simulink model "FFM_Punch"  (R2017a)
settings: Solver=ode3  StartTime=0.0  StopTime=timesteps  FixedStep=data.SIM.Ts  RelTol=1e-3  EnableMultiTasking=on
values from neighbouring files (symbols this model uses):
  data =     [dakota_config.mat]
  downshift_map = data.TCU.upshift.veh_spd_default    [Simulation_results.m]
  upshift_map = data.TCU.upshift.veh_spd_default    [Simulation_results.m]
undefined symbols (not defined in the file or in its folder): air_density, Cd, DiscIntNeverNeededParam, fr_crankshaft, fr_speed_values, g, i_FD, ICE, Low_Ratio, M_Eng_Max, M_Eng_Max_Max, M_Eng_Max_Rpm, mt2m_f, mu_Roll_C0, mu_Roll_C1, mu_Roll_C2, Mv, n_Idle_Eng, Overdrive_Ratio, Re, S_eff_drag, Ts
(part 4 of 15)

== system FFM_Punch/Vehicle/Subsystem ==
  v_veh : Inport  Tag=Controls_Lib  Description=Inp  Interpolate=off
  AddSub : Sum  Tag=Controls_Lib  Description=AddSub  Inputs=+++  CollapseDim=CollapseDim  AccumDataTypeStr=single  OutMin=OutMin  OutMax=OutMax  OutDataTypeStr=single  RndMeth=Nearest  SampleTime=SampleTime  InputSameDT=on  mask(AddSub){IconShape=rectangular, Inputs=+++, CollapseMode=All dimensions, CollapseDim=1, SampleTime=-1, InputSameDT=on, AccumDataTypeStr=single, OutMin=[], OutMax=[], OutDataTypeStr=single, LockScale=off, RndMeth=Nearest, SaturateOnIntegerOverflow=off}
      mask prompts: IconShape "Icon shape:"; Inputs "List of signs:"; CollapseMode "Sum over:"; CollapseDim "Dimension:"; SampleTime "Sample time (-1 for inherited):"; InputSameDT "Require all inputs to have the same data type"; AccumDataTypeStr "Accumulator data type:"; OutMin "Output minimum:"; OutMax "Output maximum:"; OutDataTypeStr "Output data type:"; LockScale "Lock data type settings against changes by the fixed-point tools"; RndMeth "Integer rounding mode:"; SaturateOnIntegerOverflow "Saturate on integer overflow"
      mask help:
      | Add or subtract inputs.  Specify one of the following:
      | a) string containing + or - for each input port, | for spacer between ports (e.g. ++|-|++)
      | b) scalar, >= 1, specifies the number of input ports to be summed.
      | When there is only one input port, add or subtract elements over all dimensions or one specified dimension
      mask Help: web([fileparts(which('Lib_built')) filesep 'hlp' filesep 'lib_AddSub' '.html'], '-helpbrowser')
      mask TypeOptions IconShape: IconShape
      mask TypeOptions Inputs: Inputs
      mask TypeOptions CollapseMode: CollapseMode
      mask TypeOptions CollapseDim: CollapseDim
      mask TypeOptions SampleTime: SampleTime
      mask TypeOptions InputSameDT: InputSameDT
      mask TypeOptions AccumDataTypeStr: AccumDataTypeStr
      mask TypeOptions OutMin: OutMin
      mask TypeOptions OutMax: OutMax
      mask TypeOptions OutDataTypeStr: OutDataTypeStr
      mask TypeOptions LockScale: LockScale
      mask TypeOptions RndMeth: RndMeth
      mask TypeOptions SaturateOnIntegerOverflow: SaturateOnIntegerOverflow
  Constant : Constant  Tag=Controls_Lib  Description=constant  Value=Value  OutMin=OutMin  OutMax=OutMax  OutDataTypeStr=Inherit: Inherit via back propagation  SampleTime=SampleTime  FramePeriod=FramePeriod  mask(Constant){Value=data.VEH.road_load_calc_method, VectorParams1D=on, SampleTime=-1, FramePeriod=inf, OutMin=[], OutMax=[], OutDataTypeStr=Inherit: Inherit via back propagation, LockScale=off}
      mask prompts: Value "Simulink:blkprm_prompts:ConstConstValue"; VectorParams1D "Simulink:blkprm_prompts:AllSrcsVector1D"; SampleTime "Simulink:blkprm_prompts:AllSrcBlksSampleTime"; FramePeriod "Simulink:blkprm_prompts:AllSrcBlksFramePeriod"; OutMin "Simulink:blkprm_prompts:OutputDesignMin"; OutMax "Simulink:blkprm_prompts:OutputDesignMax"; OutDataTypeStr "Simulink:blkprm_prompts:OUTPUT_UNIFIEDDATATYPE"; LockScale "Simulink:blkprm_prompts:LockScale"
      mask help: Output the constant specified by the 'Constant value' parameter.
      mask Help: web([fileparts(which('Lib_built')) filesep 'hlp' filesep 'lib_constant' '.html'], '-helpbrowser')
      mask TypeOptions Value: Value
      mask TypeOptions VectorParams1D: VectorParams1D
      mask TypeOptions SampleTime: SampleTime
      mask TypeOptions FramePeriod: FramePeriod
      mask TypeOptions OutMin: OutMin
      mask TypeOptions OutMax: OutMax
      mask TypeOptions OutDataTypeStr: OutDataTypeStr
      mask TypeOptions LockScale: LockScale
      mask DialogControl ParameterTabVar0 Prompt: Main
      mask Display: disp(get_param(gcb,'Value'))
  Constant1 : Constant  Tag=Controls_Lib  Description=constant  Value=Value  OutMin=OutMin  OutMax=OutMax  OutDataTypeStr=Inherit: Inherit via back propagation  SampleTime=SampleTime  FramePeriod=FramePeriod  mask(Constant){Value=1.5, VectorParams1D=on, SampleTime=-1, FramePeriod=inf, OutMin=[], OutMax=[], OutDataTypeStr=Inherit: Inherit via back propagation, LockScale=off}
      mask prompts: Value "Simulink:blkprm_prompts:ConstConstValue"; VectorParams1D "Simulink:blkprm_prompts:AllSrcsVector1D"; SampleTime "Simulink:blkprm_prompts:AllSrcBlksSampleTime"; FramePeriod "Simulink:blkprm_prompts:AllSrcBlksFramePeriod"; OutMin "Simulink:blkprm_prompts:OutputDesignMin"; OutMax "Simulink:blkprm_prompts:OutputDesignMax"; OutDataTypeStr "Simulink:blkprm_prompts:OUTPUT_UNIFIEDDATATYPE"; LockScale "Simulink:blkprm_prompts:LockScale"
      mask help: Output the constant specified by the 'Constant value' parameter.
      mask Help: web([fileparts(which('Lib_built')) filesep 'hlp' filesep 'lib_constant' '.html'], '-helpbrowser')
      mask TypeOptions Value: Value
      mask TypeOptions VectorParams1D: VectorParams1D
      mask TypeOptions SampleTime: SampleTime
      mask TypeOptions FramePeriod: FramePeriod
      mask TypeOptions OutMin: OutMin
      mask TypeOptions OutMax: OutMax
      mask TypeOptions OutDataTypeStr: OutDataTypeStr
      mask TypeOptions LockScale: LockScale
      mask DialogControl ParameterTabVar0 Prompt: Main
      mask Display: disp(get_param(gcb,'Value'))
  Constant2 : Constant  Tag=Controls_Lib  Description=constant  Value=Value  OutMin=OutMin  OutMax=OutMax  OutDataTypeStr=Inherit: Inherit via back propagation  SampleTime=SampleTime  FramePeriod=FramePeriod  mask(Constant){Value=data.VEH.road_load_param_A, VectorParams1D=on, SampleTime=-1, FramePeriod=inf, OutMin=[], OutMax=[], OutDataTypeStr=Inherit: Inherit via back propagation, LockScale=off}
      mask prompts: Value "Simulink:blkprm_prompts:ConstConstValue"; VectorParams1D "Simulink:blkprm_prompts:AllSrcsVector1D"; SampleTime "Simulink:blkprm_prompts:AllSrcBlksSampleTime"; FramePeriod "Simulink:blkprm_prompts:AllSrcBlksFramePeriod"; OutMin "Simulink:blkprm_prompts:OutputDesignMin"; OutMax "Simulink:blkprm_prompts:OutputDesignMax"; OutDataTypeStr "Simulink:blkprm_prompts:OUTPUT_UNIFIEDDATATYPE"; LockScale "Simulink:blkprm_prompts:LockScale"
      mask help: Output the constant specified by the 'Constant value' parameter.
      mask Help: web([fileparts(which('Lib_built')) filesep 'hlp' filesep 'lib_constant' '.html'], '-helpbrowser')
      mask TypeOptions Value: Value
      mask TypeOptions VectorParams1D: VectorParams1D
      mask TypeOptions SampleTime: SampleTime
      mask TypeOptions FramePeriod: FramePeriod
      mask TypeOptions OutMin: OutMin
      mask TypeOptions OutMax: OutMax
      mask TypeOptions OutDataTypeStr: OutDataTypeStr
      mask TypeOptions LockScale: LockScale
      mask DialogControl ParameterTabVar0 Prompt: Main
      mask Display: disp(get_param(gcb,'Value'))
  MulDiv : Product  Tag=Controls_Lib  Description=MulDiv  Inputs=**  CollapseDim=CollapseDim  OutMin=OutMin  OutMax=OutMax  OutDataTypeStr=single  SampleTime=SampleTime  InputSameDT=on  mask(MulDiv){Inputs=**, Multiplication=Element-wise(.*), CollapseMode=All dimensions, CollapseDim=1, SampleTime=-1, InputSameDT=on, OutMin=[], OutMax=[], OutDataTypeStr=single, LockScale=off, RndMeth=Floor, SaturateOnIntegerOverflow=off}
      mask prompts: Inputs "Number of inputs:"; CollapseMode "Multiply over:"; CollapseDim "Dimension:"; SampleTime "Sample time (-1 for inherited):"; InputSameDT "Require all inputs to have the same data type"; OutMin "Output minimum:"; OutMax "Output maximum:"; OutDataTypeStr "Output data type:"; LockScale "Lock output data type setting against changes by the fixed-point tools"; RndMeth "Integer rounding mode:"; SaturateOnIntegerOverflow "Saturate on integer overflow"
      mask help:
      | Multiply or divide inputs element-wise. Specify one of the following:
      |  a) * or / for each input port. For example, **/* performs the operation 'u1*u2/u3*u4'.
      |  b) scalar specifies the number of input ports to be multiplied.
      | If there is only one input port and the Multiplication parameter is set to Element-wise(.*), a single * or / collapses the input signal using the specified operation.
      mask Help: web([fileparts(which('Lib_built')) filesep 'hlp' filesep 'lib_MulDiv' '.html'], '-helpbrowser')
      mask TypeOptions Inputs: Inputs
      mask TypeOptions Multiplication: Multiplication
      mask TypeOptions CollapseMode: CollapseMode
      mask TypeOptions CollapseDim: CollapseDim
      mask TypeOptions SampleTime: SampleTime
      mask TypeOptions InputSameDT: InputSameDT
      mask TypeOptions OutMin: OutMin
      mask TypeOptions OutMax: OutMax
      mask TypeOptions OutDataTypeStr: OutDataTypeStr
      mask TypeOptions LockScale: LockScale
      mask TypeOptions RndMeth: RndMeth
      mask TypeOptions SaturateOnIntegerOverflow: SaturateOnIntegerOverflow
  RelationalOperator : RelationalOperator  Tag=Controls_Lib  Description=RelationalOperator  Operator=<  OutDataTypeStr=boolean  SampleTime=SampleTime  RndMeth=Nearest  InputSameDT=on  mask(Relational operator){Operator=<, ZeroCross=on, SampleTime=-1, InputSameDT=on, OutDataTypeStr=boolean}
      mask prompts: Operator "Relational operator:"; ZeroCross "Enable zero-crossing detection"; SampleTime "Sample time (-1 for inherited):"; InputSameDT "Require all inputs to have the same data type"; OutDataTypeStr "Output data type:"
      mask help: Applies the selected relational operator to the inputs and outputs the result. The top (or left) input corresponds to the first operand.
      mask Help: web([fileparts(which('Lib_built')) filesep 'hlp' filesep 'lib_Relational' '.html'], '-helpbrowser')
      mask TypeOptions Operator: Operator
      mask TypeOptions ZeroCross: ZeroCross
      mask TypeOptions SampleTime: SampleTime
      mask TypeOptions InputSameDT: InputSameDT
      mask TypeOptions OutDataTypeStr: OutDataTypeStr
  Rolling Resistance : Subsystem
  Signed square : Subsystem
  Sum1 : Sum  SaturateOnIntegerOverflow=on  InputSameDT=on  OutDataTypeStr=Inherit: Same as first input
  Switch : Switch  Tag=Controls_Lib  Description=Switch  Criteria=u2 ~= 0  Threshold=Threshold  OutMin=OutMin  OutMax=OutMax  OutDataTypeStr=Inherit: Inherit via back propagation  RndMeth=Zero  ZeroCross=off  SampleTime=SampleTime  InputSameDT=on  mask(Switch){Criteria=u2 ~= 0, Threshold=0.5, ZeroCross=off, SampleTime=-1, InputSameDT=on, OutMin=[], OutMax=[], OutDataTypeStr=Inherit: Inherit via back propagation, LockScale=off, RndMeth=Zero, SaturateOnIntegerOverflow=off, AllowDiffInputSizes=off}
      mask prompts: Criteria "Criteria for passing first input:"; ZeroCross "Enable zero-crossing detection"; SampleTime "Sample time (-1 for inherited):"; InputSameDT "Require all data port inputs to have the same data type"; OutMin "Output minimum:"; OutMax "Output maximum:"; OutDataTypeStr "Output data type:"; LockScale "Lock output data type setting against changes by the fixed-point tools"; RndMeth "Integer rounding mode:"; SaturateOnIntegerOverflow "Saturate on integer overflow"; AllowDiffInputSizes "Allow different data input sizes (Results in variable-size output signal)"
      mask help:
      | Pass through input 1 when input 2 is not equal to 0. Otherwise, pass through input 3.  The inputs are numbered top to bottom (or left to right). The input 1 pass-through criteria are input 2 not equal to 0;
      | The first and third input ports are data ports, and the second input port is the control port. The control port signal should always be a boolean signal.
      mask Help: web([fileparts(which('Lib_built')) filesep 'hlp' filesep 'lib_Switch' '.html'], '-helpbrowser')
      mask TypeOptions Criteria: Criteria
      mask TypeOptions Threshold: Threshold
      mask TypeOptions ZeroCross: ZeroCross
      mask TypeOptions SampleTime: SampleTime
      mask TypeOptions InputSameDT: InputSameDT
      mask TypeOptions OutMin: OutMin
      mask TypeOptions OutMax: OutMax
      mask TypeOptions OutDataTypeStr: OutDataTypeStr
      mask TypeOptions LockScale: LockScale
      mask TypeOptions RndMeth: RndMeth
      mask TypeOptions SaturateOnIntegerOverflow: SaturateOnIntegerOverflow
      mask TypeOptions AllowDiffInputSizes: AllowDiffInputSizes
  kph2ms1 : Gain  Gain=1/3.6  OutDataTypeStr=Inherit: Inherit via back propagation  ParamDataTypeStr=Inherit: Same as input
  kph2ms2 : Gain  Gain=data.VEH.road_load_param_B  OutDataTypeStr=Inherit: Inherit via back propagation  ParamDataTypeStr=Inherit: Same as input
  kph2ms3 : Gain  Gain=data.VEH.road_load_param_C  OutDataTypeStr=Inherit: Inherit via back propagation  ParamDataTypeStr=Inherit: Same as input
  F_load : Outport  Tag=Controls_Lib  Description=Out  InitialOutput=0
  wires:
  Signed square/1(Aerodynamic Drag Force) -> Sum1/1
  Rolling Resistance/1(F_RR) -> Sum1/2
  kph2ms1/1 -> Rolling Resistance/1(v_veh), Signed square/1(Vehicle Speed)
  v_veh/1 -> kph2ms2/1, MulDiv/2, MulDiv/1, kph2ms1/1
  Constant/1 -> RelationalOperator/1
  Constant1/1 -> RelationalOperator/2
  RelationalOperator/1 -> Switch/2
  Sum1/1 -> Switch/1
  Switch/1 -> F_load/1
  Constant2/1 -> AddSub/1
  kph2ms2/1 -> AddSub/2
  kph2ms3/1 -> AddSub/3
  MulDiv/1 -> kph2ms3/1
  AddSub/1 -> Switch/3

== system FFM_Punch/Controller/F02_03_03_05_Raw_Gear_Target_Auto_Mode/F02_03_03_05_01_Shift_Law_12_Contribution ==
  ts_v_vectThdAutoModDown : Inport
  ts_v_vectThdAutoModUp : Inport  Port=2
  ts_z_gearTgtFwd : Inport  Port=3
  vehest_v_frntWhl : Inport  Port=4
  Logical Operator : Logic  Operator=OR  OutDataTypeStr=boolean
  Logical Operator1 : Logic  OutDataTypeStr=boolean
  Relational Operator : RelationalOperator  OutDataTypeStr=boolean  RndMeth=Nearest  InputSameDT=on
  Relational Operator1 : RelationalOperator  OutDataTypeStr=boolean  RndMeth=Nearest  InputSameDT=on
  Relational Operator2 : RelationalOperator  OutDataTypeStr=boolean  RndMeth=Nearest  InputSameDT=on
  Selector : Selector  InputPortWidth=8  IndexOptions=Index vector (dialog)  Indices=1  OutputSizes=1
      settings: AttributesFormatString=InputPortWidth = %<InputPortWidth>\nSel. Elements = %<Elements>\nIndex Mode = %<IndexMode>
  Selector1 : Selector  InputPortWidth=8  IndexOptions=Index vector (dialog)  Indices=1  OutputSizes=1
      settings: AttributesFormatString=InputPortWidth = %<InputPortWidth>\nSel. Elements = %<Elements>\nIndex Mode = %<IndexMode>
  Switch : Switch  Criteria=u2 ~= 0  OutDataTypeStr=Inherit: Inherit via back propagation  RndMeth=Zero  SaturateOnIntegerOverflow=on  InputSameDT=on
      settings: AttributesFormatString=Criteria : %<Criteria>
  constant : Constant  OutDataTypeStr=int8
  constant1 : Constant  Value=0  OutDataTypeStr=int8
  constant2 : Constant  Value=2  OutDataTypeStr=int8
  ts_z_autoGearTgt12Inc : Outport
  wires:
  [ts_v_vectThdAutoModDown] -> Selector1/1
  [ts_v_vectThdAutoModUp] -> Selector/1
  [vehest_v_frntWhl] -> Relational Operator/1
  Selector/1 -> Relational Operator/2
  constant/1 -> Switch/1
  constant1/1 -> Switch/3
  Logical Operator/1 -> Switch/2
  Relational Operator/1 -> Logical Operator/1
  [vehest_v_frntWhl] -> Relational Operator1/1
  Selector1/1 -> Relational Operator1/2
  Logical Operator1/1 -> Logical Operator/2
  Relational Operator1/1 -> Logical Operator1/1
  Relational Operator2/1 -> Logical Operator1/2
  [ts_z_gearTgtFwd] -> Relational Operator2/1
  constant2/1 -> Relational Operator2/2
  Switch/1 -> [ts_z_autoGearTgt12Inc]
  [ts_z_autoGearTgt12Inc] -> ts_z_autoGearTgt12Inc/1
  ts_v_vectThdAutoModDown/1 -> [ts_v_vectThdAutoModDown]
  ts_v_vectThdAutoModUp/1 -> [ts_v_vectThdAutoModUp]
  ts_z_gearTgtFwd/1 -> [ts_z_gearTgtFwd]
  vehest_v_frntWhl/1 -> [vehest_v_frntWhl]

== system FFM_Punch/Controller/F02_03_03_05_Raw_Gear_Target_Auto_Mode/F02_03_03_05_02_Shift_Law_23_Contribution ==
  ts_v_vectThdAutoModDown : Inport
  ts_v_vectThdAutoModUp : Inport  Port=2
  vehest_v_frntWhl : Inport  Port=3
  ts_z_gearTgtFwd : Inport  Port=4
  Logical Operator : Logic  Operator=OR  OutDataTypeStr=boolean
  Logical Operator1 : Logic  OutDataTypeStr=boolean
  Relational Operator : RelationalOperator  OutDataTypeStr=boolean  RndMeth=Nearest  InputSameDT=on
  Relational Operator1 : RelationalOperator  OutDataTypeStr=boolean  RndMeth=Nearest  InputSameDT=on
  Relational Operator2 : RelationalOperator  OutDataTypeStr=boolean  RndMeth=Nearest  InputSameDT=on
  Selector : Selector  InputPortWidth=8  IndexOptions=Index vector (dialog)  Indices=2  OutputSizes=1
      settings: AttributesFormatString=InputPortWidth = %<InputPortWidth>\nSel. Elements = %<Elements>\nIndex Mode = %<IndexMode>
  Selector1 : Selector  InputPortWidth=8  IndexOptions=Index vector (dialog)  Indices=2  OutputSizes=1
      settings: AttributesFormatString=InputPortWidth = %<InputPortWidth>\nSel. Elements = %<Elements>\nIndex Mode = %<IndexMode>
  Switch : Switch  Criteria=u2 ~= 0  OutDataTypeStr=Inherit: Inherit via back propagation  RndMeth=Zero  SaturateOnIntegerOverflow=on  InputSameDT=on
      settings: AttributesFormatString=Criteria : %<Criteria>
  constant : Constant  OutDataTypeStr=int8
  constant1 : Constant  Value=0  OutDataTypeStr=int8
  constant2 : Constant  Value=3  OutDataTypeStr=int8
  ts_z_autoGearTgt23Inc : Outport
  wires:
  ts_z_gearTgtFwd/1 -> [ts_z_gearTgtFwd]
  vehest_v_frntWhl/1 -> [vehest_v_frntWhl]
  ts_v_vectThdAutoModUp/1 -> [ts_v_vectThdAutoModUp]
  ts_v_vectThdAutoModDown/1 -> [ts_v_vectThdAutoModDown]
  [ts_v_vectThdAutoModDown] -> Selector1/1
  [ts_v_vectThdAutoModUp] -> Selector/1
  [vehest_v_frntWhl] -> Relational Operator/1
  Selector/1 -> Relational Operator/2
  constant/1 -> Switch/1
  constant1/1 -> Switch/3
  Logical Operator/1 -> Switch/2
  Relational Operator/1 -> Logical Operator/1
  [vehest_v_frntWhl] -> Relational Operator1/1
  Selector1/1 -> Relational Operator1/2
  Logical Operator1/1 -> Logical Operator/2
  Relational Operator1/1 -> Logical Operator1/1
  Relational Operator2/1 -> Logical Operator1/2
  [ts_z_gearTgtFwd] -> Relational Operator2/1
  constant2/1 -> Relational Operator2/2
  Switch/1 -> [ts_z_autoGearTgt23Inc]
  [ts_z_autoGearTgt23Inc] -> ts_z_autoGearTgt23Inc/1

== system FFM_Punch/Controller/F02_03_03_05_Raw_Gear_Target_Auto_Mode/F02_03_03_05_03_Shift_Law_34_Contribution ==
  ts_v_vectThdAutoModDown : Inport
  ts_v_vectThdAutoModUp : Inport  Port=2
  vehest_v_frntWhl : Inport  Port=3
  ts_z_gearTgtFwd : Inport  Port=4
  Logical Operator : Logic  Operator=OR  OutDataTypeStr=boolean
  Logical Operator1 : Logic  OutDataTypeStr=boolean
  Relational Operator : RelationalOperator  OutDataTypeStr=boolean  RndMeth=Nearest  InputSameDT=on
  Relational Operator1 : RelationalOperator  OutDataTypeStr=boolean  RndMeth=Nearest  InputSameDT=on
  Relational Operator2 : RelationalOperator  OutDataTypeStr=boolean  RndMeth=Nearest  InputSameDT=on
  Selector : Selector  InputPortWidth=8  IndexOptions=Index vector (dialog)  Indices=3  OutputSizes=1
      settings: AttributesFormatString=InputPortWidth = %<InputPortWidth>\nSel. Elements = %<Elements>\nIndex Mode = %<IndexMode>
  Selector1 : Selector  InputPortWidth=8  IndexOptions=Index vector (dialog)  Indices=3  OutputSizes=1
      settings: AttributesFormatString=InputPortWidth = %<InputPortWidth>\nSel. Elements = %<Elements>\nIndex Mode = %<IndexMode>
  Switch : Switch  Criteria=u2 ~= 0  OutDataTypeStr=Inherit: Inherit via back propagation  RndMeth=Zero  SaturateOnIntegerOverflow=on  InputSameDT=on
      settings: AttributesFormatString=Criteria : %<Criteria>
  constant : Constant  OutDataTypeStr=int8
  constant1 : Constant  Value=0  OutDataTypeStr=int8
  constant2 : Constant  Value=4  OutDataTypeStr=int8
  ts_z_autoGearTgt34Inc : Outport
  wires:
  ts_z_gearTgtFwd/1 -> [ts_z_gearTgtFwd]
  vehest_v_frntWhl/1 -> [vehest_v_frntWhl]
  ts_v_vectThdAutoModUp/1 -> [ts_v_vectThdAutoModUp]
  ts_v_vectThdAutoModDown/1 -> [ts_v_vectThdAutoModDown]
  [ts_v_vectThdAutoModDown] -> Selector1/1
  [ts_v_vectThdAutoModUp] -> Selector/1
  [vehest_v_frntWhl] -> Relational Operator/1
  Selector/1 -> Relational Operator/2
  constant/1 -> Switch/1
  constant1/1 -> Switch/3
  Logical Operator/1 -> Switch/2
  Relational Operator/1 -> Logical Operator/1
  [vehest_v_frntWhl] -> Relational Operator1/1
  Selector1/1 -> Relational Operator1/2
  Logical Operator1/1 -> Logical Operator/2
  Relational Operator1/1 -> Logical Operator1/1
  Relational Operator2/1 -> Logical Operator1/2
  [ts_z_gearTgtFwd] -> Relational Operator2/1
  constant2/1 -> Relational Operator2/2
  Switch/1 -> [ts_z_autoGearTgt34Inc]
  [ts_z_autoGearTgt34Inc] -> ts_z_autoGearTgt34Inc/1

== system FFM_Punch/Controller/F02_03_03_05_Raw_Gear_Target_Auto_Mode/F02_03_03_05_04_Shift_Law_45_Contribution ==
  ts_v_vectThdAutoModDown : Inport
  ts_v_vectThdAutoModUp : Inport  Port=2
  vehest_v_frntWhl : Inport  Port=3
  ts_z_gearTgtFwd : Inport  Port=4
  Logical Operator : Logic  Operator=OR  OutDataTypeStr=boolean
  Logical Operator1 : Logic  OutDataTypeStr=boolean
  Relational Operator : RelationalOperator  OutDataTypeStr=boolean  RndMeth=Nearest  InputSameDT=on
  Relational Operator1 : RelationalOperator  OutDataTypeStr=boolean  RndMeth=Nearest  InputSameDT=on
  Relational Operator2 : RelationalOperator  OutDataTypeStr=boolean  RndMeth=Nearest  InputSameDT=on
  Selector : Selector  InputPortWidth=8  IndexOptions=Index vector (dialog)  Indices=4  OutputSizes=1
      settings: AttributesFormatString=InputPortWidth = %<InputPortWidth>\nSel. Elements = %<Elements>\nIndex Mode = %<IndexMode>
  Selector1 : Selector  InputPortWidth=8  IndexOptions=Index vector (dialog)  Indices=4  OutputSizes=1
      settings: AttributesFormatString=InputPortWidth = %<InputPortWidth>\nSel. Elements = %<Elements>\nIndex Mode = %<IndexMode>
  Switch : Switch  Criteria=u2 ~= 0  OutDataTypeStr=Inherit: Inherit via back propagation  RndMeth=Zero  SaturateOnIntegerOverflow=on  InputSameDT=on
      settings: AttributesFormatString=Criteria : %<Criteria>
  constant : Constant  OutDataTypeStr=int8
  constant1 : Constant  Value=0  OutDataTypeStr=int8
  constant2 : Constant  Value=5  OutDataTypeStr=int8
  ts_z_autoGearTgt45Inc : Outport
  wires:
  ts_z_gearTgtFwd/1 -> [ts_z_gearTgtFwd]
  vehest_v_frntWhl/1 -> [vehest_v_frntWhl]
  ts_v_vectThdAutoModUp/1 -> [ts_v_vectThdAutoModUp]
  ts_v_vectThdAutoModDown/1 -> [ts_v_vectThdAutoModDown]
  [ts_v_vectThdAutoModDown] -> Selector1/1
  [ts_v_vectThdAutoModUp] -> Selector/1
  [vehest_v_frntWhl] -> Relational Operator/1
  Selector/1 -> Relational Operator/2
  constant/1 -> Switch/1
  constant1/1 -> Switch/3
  Logical Operator/1 -> Switch/2
  Relational Operator/1 -> Logical Operator/1
  [vehest_v_frntWhl] -> Relational Operator1/1
  Selector1/1 -> Relational Operator1/2
  Logical Operator1/1 -> Logical Operator/2
  Relational Operator1/1 -> Logical Operator1/1
  Relational Operator2/1 -> Logical Operator1/2
  [ts_z_gearTgtFwd] -> Relational Operator2/1
  constant2/1 -> Relational Operator2/2
  Switch/1 -> [ts_z_autoGearTgt45Inc]
  [ts_z_autoGearTgt45Inc] -> ts_z_autoGearTgt45Inc/1

== system FFM_Punch/Controller/F02_03_03_05_Raw_Gear_Target_Auto_Mode/F02_03_03_05_05_Shift_Law_56_Contribution ==
  ts_v_vectThdAutoModDown : Inport
  ts_v_vectThdAutoModUp : Inport  Port=2
  vehest_v_frntWhl : Inport  Port=3
  ts_z_gearTgtFwd : Inport  Port=4
  Logical Operator : Logic  Operator=OR  OutDataTypeStr=boolean
  Logical Operator1 : Logic  OutDataTypeStr=boolean
  Relational Operator : RelationalOperator  OutDataTypeStr=boolean  RndMeth=Nearest  InputSameDT=on
  Relational Operator1 : RelationalOperator  OutDataTypeStr=boolean  RndMeth=Nearest  InputSameDT=on
  Relational Operator2 : RelationalOperator  OutDataTypeStr=boolean  RndMeth=Nearest  InputSameDT=on
  Selector : Selector  InputPortWidth=8  IndexOptions=Index vector (dialog)  Indices=5  OutputSizes=1
      settings: AttributesFormatString=InputPortWidth = %<InputPortWidth>\nSel. Elements = %<Elements>\nIndex Mode = %<IndexMode>
  Selector1 : Selector  InputPortWidth=8  IndexOptions=Index vector (dialog)  Indices=5  OutputSizes=1
      settings: AttributesFormatString=InputPortWidth = %<InputPortWidth>\nSel. Elements = %<Elements>\nIndex Mode = %<IndexMode>
  Switch : Switch  Criteria=u2 ~= 0  OutDataTypeStr=Inherit: Inherit via back propagation  RndMeth=Zero  SaturateOnIntegerOverflow=on  InputSameDT=on
      settings: AttributesFormatString=Criteria : %<Criteria>
  constant : Constant  OutDataTypeStr=int8
  constant1 : Constant  Value=0  OutDataTypeStr=int8
  constant2 : Constant  Value=6  OutDataTypeStr=int8
  ts_z_autoGearTgt56Inc : Outport
  wires:
  ts_z_gearTgtFwd/1 -> [ts_z_gearTgtFwd]
  vehest_v_frntWhl/1 -> [vehest_v_frntWhl]
  ts_v_vectThdAutoModUp/1 -> [ts_v_vectThdAutoModUp]
  ts_v_vectThdAutoModDown/1 -> [ts_v_vectThdAutoModDown]
  [ts_v_vectThdAutoModDown] -> Selector1/1
  [ts_v_vectThdAutoModUp] -> Selector/1
  [vehest_v_frntWhl] -> Relational Operator/1
  Selector/1 -> Relational Operator/2
  constant/1 -> Switch/1
  constant1/1 -> Switch/3
  Logical Operator/1 -> Switch/2
  Relational Operator/1 -> Logical Operator/1
  [vehest_v_frntWhl] -> Relational Operator1/1
  Selector1/1 -> Relational Operator1/2
  Logical Operator1/1 -> Logical Operator/2
  Relational Operator1/1 -> Logical Operator1/1
  Relational Operator2/1 -> Logical Operator1/2
  [ts_z_gearTgtFwd] -> Relational Operator2/1
  constant2/1 -> Relational Operator2/2
  Switch/1 -> [ts_z_autoGearTgt56Inc]
  [ts_z_autoGearTgt56Inc] -> ts_z_autoGearTgt56Inc/1

== system FFM_Punch/Controller/F02_03_03_05_Raw_Gear_Target_Auto_Mode/F02_03_03_05_06_Shift_Law_67_Contribution ==
  ts_v_vectThdAutoModDown : Inport
  ts_v_vectThdAutoModUp : Inport  Port=2
  vehest_v_frntWhl : Inport  Port=3
  ts_z_gearTgtFwd : Inport  Port=4
  Logical Operator : Logic  Operator=OR  OutDataTypeStr=boolean
  Logical Operator1 : Logic  OutDataTypeStr=boolean
  Relational Operator : RelationalOperator  OutDataTypeStr=boolean  RndMeth=Nearest  InputSameDT=on
  Relational Operator1 : RelationalOperator  OutDataTypeStr=boolean  RndMeth=Nearest  InputSameDT=on
  Relational Operator2 : RelationalOperator  OutDataTypeStr=boolean  RndMeth=Nearest  InputSameDT=on
  Selector : Selector  InputPortWidth=8  IndexOptions=Index vector (dialog)  Indices=6  OutputSizes=1
      settings: AttributesFormatString=InputPortWidth = %<InputPortWidth>\nSel. Elements = %<Elements>\nIndex Mode = %<IndexMode>
  Selector1 : Selector  InputPortWidth=8  IndexOptions=Index vector (dialog)  Indices=6  OutputSizes=1
      settings: AttributesFormatString=InputPortWidth = %<InputPortWidth>\nSel. Elements = %<Elements>\nIndex Mode = %<IndexMode>
  Switch : Switch  Criteria=u2 ~= 0  OutDataTypeStr=Inherit: Inherit via back propagation  RndMeth=Zero  SaturateOnIntegerOverflow=on  InputSameDT=on
      settings: AttributesFormatString=Criteria : %<Criteria>
  constant : Constant  OutDataTypeStr=int8
  constant1 : Constant  Value=0  OutDataTypeStr=int8
  constant2 : Constant  Value=7  OutDataTypeStr=int8
  ts_z_autoGearTgt67Inc : Outport
  wires:
  ts_z_gearTgtFwd/1 -> [ts_z_gearTgtFwd]
  vehest_v_frntWhl/1 -> [vehest_v_frntWhl]
  ts_v_vectThdAutoModUp/1 -> [ts_v_vectThdAutoModUp]
  ts_v_vectThdAutoModDown/1 -> [ts_v_vectThdAutoModDown]
  [ts_v_vectThdAutoModDown] -> Selector1/1
  [ts_v_vectThdAutoModUp] -> Selector/1
  [vehest_v_frntWhl] -> Relational Operator/1
  Selector/1 -> Relational Operator/2
  constant/1 -> Switch/1
  constant1/1 -> Switch/3
  Logical Operator/1 -> Switch/2
  Relational Operator/1 -> Logical Operator/1
  [vehest_v_frntWhl] -> Relational Operator1/1
  Selector1/1 -> Relational Operator1/2
  Logical Operator1/1 -> Logical Operator/2
  Relational Operator1/1 -> Logical Operator1/1
  Relational Operator2/1 -> Logical Operator1/2
  [ts_z_gearTgtFwd] -> Relational Operator2/1
  constant2/1 -> Relational Operator2/2
  Switch/1 -> [ts_z_autoGearTgt67Inc]
  [ts_z_autoGearTgt67Inc] -> ts_z_autoGearTgt67Inc/1

== system FFM_Punch/Controller/F02_03_03_05_Raw_Gear_Target_Auto_Mode/F02_03_03_05_07_Shift_Law_78_Contribution ==
  ts_v_vectThdAutoModDown : Inport
  ts_v_vectThdAutoModUp : Inport  Port=2
  vehest_v_frntWhl : Inport  Port=3
  ts_z_gearTgtFwd : Inport  Port=4
  Logical Operator : Logic  Operator=OR  OutDataTypeStr=boolean
  Logical Operator1 : Logic  OutDataTypeStr=boolean
  Relational Operator : RelationalOperator  OutDataTypeStr=boolean  RndMeth=Nearest  InputSameDT=on
  Relational Operator1 : RelationalOperator  OutDataTypeStr=boolean  RndMeth=Nearest  InputSameDT=on
  Relational Operator2 : RelationalOperator  OutDataTypeStr=boolean  RndMeth=Nearest  InputSameDT=on
  Selector : Selector  InputPortWidth=8  IndexOptions=Index vector (dialog)  Indices=7  OutputSizes=1
      settings: AttributesFormatString=InputPortWidth = %<InputPortWidth>\nSel. Elements = %<Elements>\nIndex Mode = %<IndexMode>
  Selector1 : Selector  InputPortWidth=8  IndexOptions=Index vector (dialog)  Indices=7  OutputSizes=1
      settings: AttributesFormatString=InputPortWidth = %<InputPortWidth>\nSel. Elements = %<Elements>\nIndex Mode = %<IndexMode>
  Switch : Switch  Criteria=u2 ~= 0  OutDataTypeStr=Inherit: Inherit via back propagation  RndMeth=Zero  SaturateOnIntegerOverflow=on  InputSameDT=on
      settings: AttributesFormatString=Criteria : %<Criteria>
  constant : Constant  OutDataTypeStr=int8
  constant1 : Constant  Value=0  OutDataTypeStr=int8
  constant2 : Constant  Value=8  OutDataTypeStr=int8
  ts_z_autoGearTgt78Inc : Outport
  wires:
  [ts_z_autoGearTgt78Inc] -> ts_z_autoGearTgt78Inc/1
  Switch/1 -> [ts_z_autoGearTgt78Inc]
  constant2/1 -> Relational Operator2/2
  [ts_z_gearTgtFwd] -> Relational Operator2/1
  Relational Operator2/1 -> Logical Operator1/2
  Relational Operator1/1 -> Logical Operator1/1
  Logical Operator1/1 -> Logical Operator/2
  Selector1/1 -> Relational Operator1/2
  [vehest_v_frntWhl] -> Relational Operator1/1
  Relational Operator/1 -> Logical Operator/1
  Logical Operator/1 -> Switch/2
  constant1/1 -> Switch/3
  constant/1 -> Switch/1
  Selector/1 -> Relational Operator/2
  [vehest_v_frntWhl] -> Relational Operator/1
  [ts_v_vectThdAutoModUp] -> Selector/1
  [ts_v_vectThdAutoModDown] -> Selector1/1
  ts_v_vectThdAutoModDown/1 -> [ts_v_vectThdAutoModDown]
  ts_v_vectThdAutoModUp/1 -> [ts_v_vectThdAutoModUp]
  vehest_v_frntWhl/1 -> [vehest_v_frntWhl]
  ts_z_gearTgtFwd/1 -> [ts_z_gearTgtFwd]

== system FFM_Punch/Controller/F02_03_03_05_Raw_Gear_Target_Auto_Mode/F02_03_03_05_08_Shift_Law_89_Contribution ==
  ts_v_vectThdAutoModDown : Inport
  ts_v_vectThdAutoModUp : Inport  Port=2
  vehest_v_frntWhl : Inport  Port=3
  ts_z_gearTgtFwd : Inport  Port=4
  Logical Operator : Logic  Operator=OR  OutDataTypeStr=boolean
  Logical Operator1 : Logic  OutDataTypeStr=boolean
  Relational Operator : RelationalOperator  OutDataTypeStr=boolean  RndMeth=Nearest  InputSameDT=on
  Relational Operator1 : RelationalOperator  OutDataTypeStr=boolean  RndMeth=Nearest  InputSameDT=on
  Relational Operator2 : RelationalOperator  OutDataTypeStr=boolean  RndMeth=Nearest  InputSameDT=on
  Selector : Selector  InputPortWidth=8  IndexOptions=Index vector (dialog)  Indices=8  OutputSizes=1
      settings: AttributesFormatString=InputPortWidth = %<InputPortWidth>\nSel. Elements = %<Elements>\nIndex Mode = %<IndexMode>
  Selector1 : Selector  InputPortWidth=8  IndexOptions=Index vector (dialog)  Indices=8  OutputSizes=1
      settings: AttributesFormatString=InputPortWidth = %<InputPortWidth>\nSel. Elements = %<Elements>\nIndex Mode = %<IndexMode>
  Switch : Switch  Criteria=u2 ~= 0  OutDataTypeStr=Inherit: Inherit via back propagation  RndMeth=Zero  SaturateOnIntegerOverflow=on  InputSameDT=on
      settings: AttributesFormatString=Criteria : %<Criteria>
  constant : Constant  OutDataTypeStr=int8
  constant1 : Constant  Value=0  OutDataTypeStr=int8
  constant2 : Constant  Value=9  OutDataTypeStr=int8
  ts_z_autoGearTgt89Inc : Outport
  wires:
  [ts_z_autoGearTgt89Inc] -> ts_z_autoGearTgt89Inc/1
  ts_z_gearTgtFwd/1 -> [ts_z_gearTgtFwd]
  vehest_v_frntWhl/1 -> [vehest_v_frntWhl]
  ts_v_vectThdAutoModUp/1 -> [ts_v_vectThdAutoModUp]
  ts_v_vectThdAutoModDown/1 -> [ts_v_vectThdAutoModDown]
  [ts_v_vectThdAutoModDown] -> Selector1/1
  [ts_v_vectThdAutoModUp] -> Selector/1
  [vehest_v_frntWhl] -> Relational Operator/1
  Selector/1 -> Relational Operator/2
  constant/1 -> Switch/1
  constant1/1 -> Switch/3
  Logical Operator/1 -> Switch/2
  Relational Operator/1 -> Logical Operator/1
  [vehest_v_frntWhl] -> Relational Operator1/1
  Selector1/1 -> Relational Operator1/2
  Logical Operator1/1 -> Logical Operator/2
  Relational Operator1/1 -> Logical Operator1/1
  Relational Operator2/1 -> Logical Operator1/2
  [ts_z_gearTgtFwd] -> Relational Operator2/1
  constant2/1 -> Relational Operator2/2
  Switch/1 -> [ts_z_autoGearTgt89Inc]
